simulink model "Sistema_Sencillo"  (R2017b)
settings: Solver=FixedStepAuto  StartTime=0.0  StopTime=10.0  FixedStep=0.01  RelTol=1e-3
values from neighbouring files (symbols this model uses):
  B = 20    [Sistema_Complejo.m]    (also in Sistema_Sencillo.m)
  K = 491.1    [Sistema_Sencillo.m]
  M = 5.23    [Sistema_Sencillo.m]
  ST = 1    [Sistema_Complejo.m]    (also in Sistema_Sencillo.m)
  V0 = 0    [Sistema_Sencillo.m]
  VF = 100    [Sistema_Sencillo.m]
  VI = 0    [Sistema_Complejo.m]    (also in Sistema_Sencillo.m)
  X0 = 0    [Sistema_Sencillo.m]
settings Model: Creator=carlos  LastModifiedBy=Wilmer
settings CodeAppCC: StateflowObjectComments=on

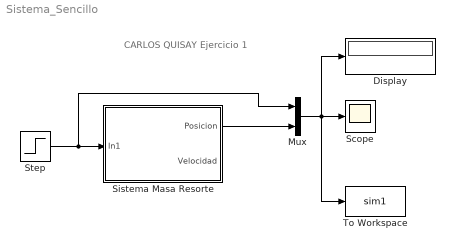
== system Sistema_Sencillo ==
  note: CARLOS QUISAY
      | Ejercicio 1
  Display : Display
  Mux : Mux  Inputs=2
  Scope : Scope
  Sistema Masa Resorte : Subsystem
  Step : Step  Time=ST  Before=VI  After=VF  SampleTime=0
  To Workspace : ToWorkspace  VariableName=sim1  SampleTime=-1
  wires:
  Step/1 -> Mux/1, Sistema Masa Resorte/1(In1)
  Sistema Masa Resorte/1(Posicion) -> Mux/2
  Mux/1 -> To Workspace/1, Display/1, Scope/1

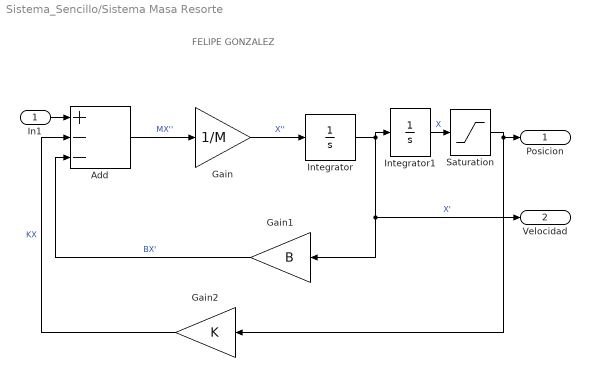
== system Sistema_Sencillo/Sistema Masa Resorte ==
  note: FELIPE GONZALEZ
  In1 : Inport
  Add : Sum  Inputs=+--
  Gain : Gain  Gain=1/M
  Gain1 : Gain  Gain=B
  Gain2 : Gain  Gain=K
  Integrator : Integrator  InitialCondition=V0
  Integrator1 : Integrator  InitialCondition=X0
  Saturation : Saturate  UpperLimit=0.25  LowerLimit=0
  Posicion : Outport
  Velocidad : Outport  Port=2
  wires:
  In1/1 -> Add/1
  Integrator/1 -> Velocidad/1, Gain1/1, Integrator1/1  "X'"
  Gain1/1 -> Add/3  "BX'"
  Gain2/1 -> Add/2  "KX"
  Integrator1/1 -> Saturation/1  "X"
  Gain/1 -> Integrator/1  "X''"
  Add/1 -> Gain/1  "MX''"
  Saturation/1 -> Posicion/1, Gain2/1
